simulink model "tcp"  (R2021b)
settings: Solver=VariableStepAuto  StartTime=0.0  StopTime=10.0  RelTol=1e-3
libraries: instrumentlib x2
settings Model: Creator=Duy  LastModifiedBy=Duy

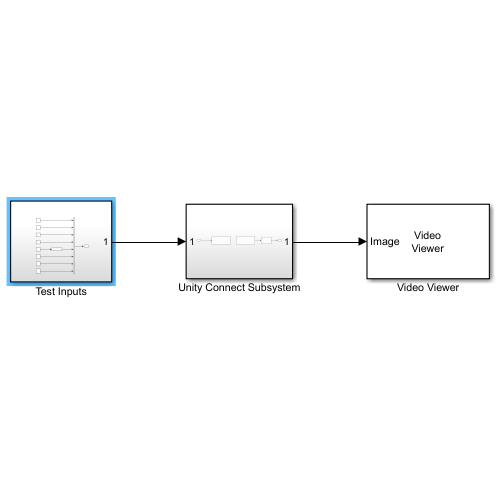
[thumbnail: Simulink's stored preview of the top-level diagram]
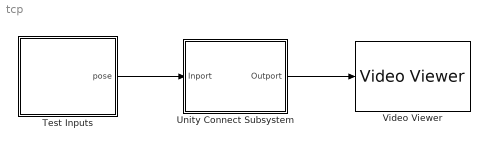
== system tcp ==
  Test Inputs : Subsystem
  Unity Connect Subsystem : Subsystem  Priority=2
  Video Viewer : VideoViewer  FigPos=[2190 892 646 535]
  wires:
  Test Inputs/1(pose) -> Unity Connect Subsystem/1(Inport)
  Unity Connect Subsystem/1(Outport) -> Video Viewer/1

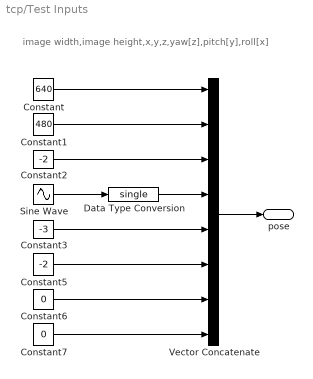
== system tcp/Test Inputs ==
  note: image width,image height,x,y,z,yaw[z],pitch[y],roll[x]
  Constant : Constant  Value=640  OutDataTypeStr=single
  Constant1 : Constant  Value=480  OutDataTypeStr=single
  Constant2 : Constant  Value=-2  OutDataTypeStr=single
  Constant3 : Constant  Value=-3  OutDataTypeStr=single
  Constant5 : Constant  Value=-2  OutDataTypeStr=single
  Constant6 : Constant  Value=0  OutDataTypeStr=single
  Constant7 : Constant  Value=0  OutDataTypeStr=single
  Data Type Conversion : DataTypeConversion  OutDataTypeStr=single
  Sine Wave : Sin  SampleTime=0.01
  Vector Concatenate : Concatenate  NumInputs=8
  pose : Outport
  wires:
  Constant1/1 -> Vector Concatenate/2
  Vector Concatenate/1 -> pose/1
  Constant/1 -> Vector Concatenate/1
  Constant2/1 -> Vector Concatenate/3
  Constant3/1 -> Vector Concatenate/5
  Data Type Conversion/1 -> Vector Concatenate/4
  Constant5/1 -> Vector Concatenate/6
  Constant6/1 -> Vector Concatenate/7
  Constant7/1 -> Vector Concatenate/8
  Sine Wave/1 -> Data Type Conversion/1

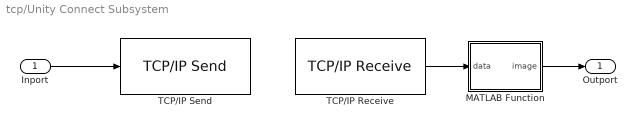
== system tcp/Unity Connect Subsystem ==
  Inport : Inport
  MATLAB Function : MATLAB Function  TreatAsAtomicUnit=on
  TCP/IP Receive : instrumentlib/TCP//IP Receive  Description=receive data from Unity, must set priorty to 2  Priority=2  Host=127.0.0.1  Port=55001  DataSize="[640  480    3]"  DataType=uint8  ASCIIFormatting=%f  Terminator=LF  CustomTerminator=10  ByteOrder=big-endian  EnableBlockingMode=on  Timeout=20  SampleTime=-1  SimulateUsing=Interpreted execution
  TCP/IP Send : instrumentlib/TCP//IP Send  Description=send data to Unity, must set priority to 1  Priority=1  Host=127.0.0.1  Port=55001  ByteOrder=little-endian  EnableBlockingMode=on  Timeout=10  TransferDelay=off  SimulateUsing=Interpreted execution
  Outport : Outport
  wires:
  TCP/IP Receive/1 -> MATLAB Function/1(data)
  Inport/1 -> TCP/IP Send/1
  MATLAB Function/1(image) -> Outport/1

== matlab function tcp/Unity Connect Subsystem/MATLAB Function ==
  data: data input; image output
function image = fcn(data)
x = size(data);
width = x(1);
height = x(2);
temp = reshape(data, [3, width * height]);
image = imrotate(reshape(temp', [width, height, 3]), 90);
